simulink library "PAYLOAD_MASTER"  (Simulink 8.8)
settings: Solver=ode45  StartTime=0.0  StopTime=10.0  RelTol=1e-3  EnableMultiTasking=on
libraries: cdsEpicsOut x123, cdsFilt x55, cdsTP x42, cdsFiltCtrl x33, cdsEpicsIn x31, cdsMuxMatrix x17, cdsEpicsBinIn x17, VIS_LIB x13, PAYLOAD_MASTER x13, cdsRms x8, simulink x6, cdsEpicsStringIn x6
(part 3 of 12)

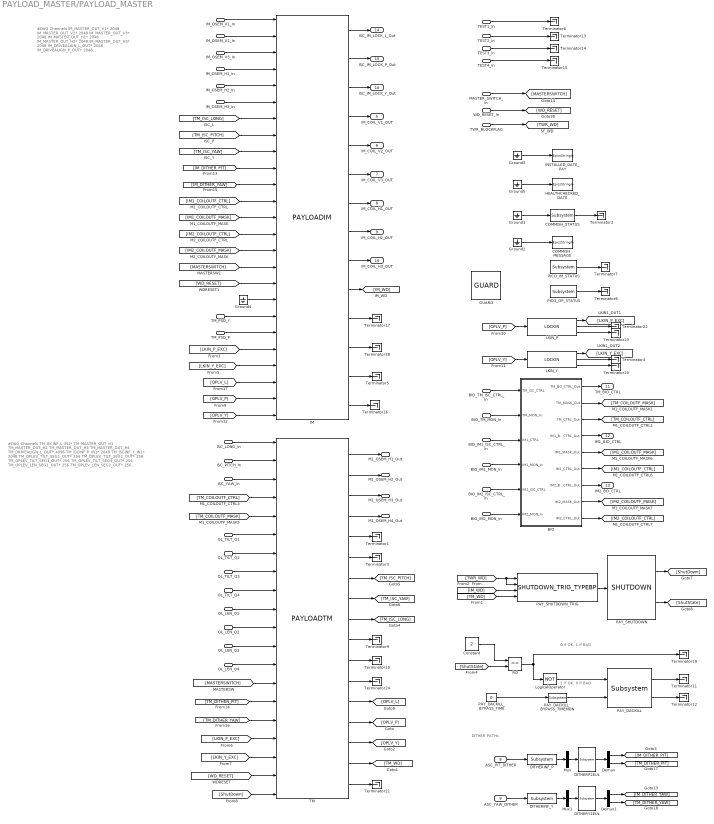
== system PAYLOAD_MASTER/PAYLOAD_MASTER ==
  note: 0 if OK, 1 if BAD
  note: 1 if OK, 0 if BAD
  note: #DAQ Channels
      | IM_MASTER_OUT_V1* 2048
      | IM_MASTER_OUT_V2* 2048
      | IM_MASTER_OUT_V3* 2048
      | IM_MASTER_OUT_H1* 2048
      | IM_MASTER_OUT_H2* 2048
      | IM_MASTER_OUT_H3* 2048
      | IM_DRIVEALIGN_L_OUT* 2048
      | IM_DRIVEALIGN_P_OUT* 2048
      | IM_DRIVEALIGN_Y_OUT* 2048
      | IM_CAL_LINE_OUT* 512
      | IM_OLDAMP_P_OUT* 256
      | IM_OLDAMP_Y_OUT* 256
      | IM_OSEMINF_V1_OUT* 256
      | IM_OSEMINF_V2_OUT* 256
      | IM_OSEMINF_V3_OUT* 256
      | IM_OSEMINF_H1_OUT* 256
      | IM_OSEMINF_H2_OUT* 256
      | IM_OSEMINF_H3_OUT* 256
  note: #DAQ Channels
      | TM_ISCINF_L_IN1*
      | TM_MASTER_OUT_H1
      | TM_MASTER_OUT_H2
      | TM_MASTER_OUT_H3
      | TM_MASTER_OUT_H4
      |
      | TM_DRIVEALIGN_L_OUT* 4096
      |
      | TM_ISCINF_P_IN1* 2048
      | TM_ISCINF_Y_IN1* 2048
      |
      | TM_OPLEV_TILT_SEG1_OUT* 256
      | TM_OPLEV_TILT_SEG2_OUT* 256
      | TM_OPLEV_TILT_SEG3_OUT* 256
      | TM_OPLEV_TILT_SEG4_OUT* 256
      | TM_OPLEV_LEN_SEG1_OUT* 256
      | TM_OPLEV_LEN_SEG2_OUT* 256
      | TM_OPLEV_LEN_SEG3_OUT* 256
      | TM_OPLEV_LEN_SEG4_OUT* 256
      |
      | TM_OPLEV_TILT_PIT_OUT* 256
      | TM_OPLEV_TILT_YAW_OUT* 256
      | TM_OPLEV_TILT_SUM_OUT* 256
      | TM_OPLEV_LEN_PIT_OUT* 256
      | TM_OPLEV_LEN_YAW_OUT* 256
      | TM_OPLEV_LEN_SUM_OUT* 256
  note: DITHER PATHs
  ISC_LONG_In : Inport
  ISC_PITCH_In : Inport  Port=2
  ISC_YAW_In : Inport  Port=3
  OL_TILT_Q1 : Inport  Port=4
  OL_TILT_Q2 : Inport  Port=5
  OL_TILT_Q3 : Inport  Port=6
  OL_TILT_Q4 : Inport  Port=7
  ASC_PIT_DITHER : Inport  Port=8
  ASC_YAW_DITHER : Inport  Port=9
  IM_OSEM_V1_In : Inport  Port=10
  IM_OSEM_V2_In : Inport  Port=11
  IM_OSEM_V3_In : Inport  Port=12
  IM_OSEM_H1_In : Inport  Port=13
  IM_OSEM_H2_In : Inport  Port=14
  IM_OSEM_H3_In : Inport  Port=15
  TEST1_In : Inport  Port=16
  TEST2_In : Inport  Port=17
  TEST3_In : Inport  Port=18
  TEST4_In : Inport  Port=19
  OL_LEN_Q1 : Inport  Port=20
  OL_LEN_Q2 : Inport  Port=21
  OL_LEN_Q3 : Inport  Port=22
  OL_LEN_Q4 : Inport  Port=23
  BIO_TM_ISC_CTRL_In : Inport  Port=24
  BIO_IM1_ISC_CTRL_In : Inport  Port=25
  BIO_IM2_ISC_CTRL_In : Inport  Port=26
  BIO_TM_MON_In : Inport  Port=27
  BIO_IM1_MON_In : Inport  Port=28
  BIO_IM2_MON_In : Inport  Port=29
  TM_PSD_P : Inport  Port=30
  TM_PSD_Y : Inport  Port=31
  MASTER_SWITCH_In : Inport  Port=32
  WD_RESET_In : Inport  Port=33
  TWR_BLOCKFLAG : Inport  Port=34
  BIO : Subsystem
  COMMISH_MESSAGE : cdsEpicsStringIn/EpicsStringIn  Tag=cdsEpicsStringIn  Description=cdsEpicsStringIn
      settings: AttributesFormatString=%<Tag>
  COMMISH_STATUS : cdsEpicsBinIn/Subsystem  Tag=cdsEpicsBinIn  Description=|
      | Purpose:                                                                            
      | Create an EPICS binary (0 or 1) input channel to the FE realtime controls.          
      |                                                                                     
      | Operation:                                                                          
      | Outputs value from an EPICS ai record. Value is binary input (bi Epics record type).
      |                                                                                     
      | Usage:                                                                              
      | Name the part with the desired EPICS channel name.
      settings: AttributesFormatString=%<Tag>
  Constant : Constant  Value=2
  DITHERINF_P : cdsFilt/Subsystem  Tag=cdsFilt  Description=|
      | Purpose:                                                                                                                                                                                                                                  
      | Standard CDS IIR filter module.                                                                                                                                                                                                           
      |                                                                                                                                                                                                                                           
      | Operation:                                                                                                                                                                                                                                
      | Consists of 10 second order section IIR filters, plus a ramped gain stage. In FE code, also provides pre-defined test points and excitation channel inputs. The filter coefficients are defined in the LIGO system using the 'foton' tool.
      |                                                                                                                                                                                                                                           
      | Usage:                                                                                                                                                                                                                                    
      | Name the part with the desired filter module name.
      settings: AttributesFormatString=%<Tag>
  DITHERINF_Y : cdsFilt/Subsystem  Tag=cdsFilt  Description=|
      | Purpose:                                                                                                                                                                                                                                  
      | Standard CDS IIR filter module.                                                                                                                                                                                                           
      |                                                                                                                                                                                                                                           
      | Operation:                                                                                                                                                                                                                                
      | Consists of 10 second order section IIR filters, plus a ramped gain stage. In FE code, also provides pre-defined test points and excitation channel inputs. The filter coefficients are defined in the LIGO system using the 'foton' tool.
      |                                                                                                                                                                                                                                           
      | Usage:                                                                                                                                                                                                                                    
      | Name the part with the desired filter module name.
      settings: AttributesFormatString=%<Tag>
  DITHERP2EUL : cdsMuxMatrix/Subsystem  Tag=cdsMuxMatrix  Description=Any size matrix. Inputs and outputs must be connected using Mux and Demux parts.
      settings: AttributesFormatString=%<Tag>
  DITHERY2EUL : cdsMuxMatrix/Subsystem  Tag=cdsMuxMatrix  Description=Any size matrix. Inputs and outputs must be connected using Mux and Demux parts.
      settings: AttributesFormatString=%<Tag>
  Demux : Demux  Outputs=2
  Demux1 : Demux  Outputs=2
  GUARD : ISC_common/GUARD
  Ground{1..5} (5 alike) : Ground
  HEALTHCHECKED_DATE : cdsEpicsStringIn/EpicsStringIn  Tag=cdsEpicsStringIn  Description=cdsEpicsStringIn
      settings: AttributesFormatString=%<Tag>
  IM : PAYLOAD_MASTER/PAYLOADIM  Description=SIXOSEMSTAGE_FACE_MASTER
  INSTALLED_DATE_PAY : cdsEpicsStringIn/EpicsStringIn  Tag=cdsEpicsStringIn  Description=cdsEpicsStringIn
      settings: AttributesFormatString=%<Tag>
  LKIN_P : lockin/LOCKIN  Description=ADL=LOCKIN.adl
      settings: AttributesFormatString=%<Tag>
  LKIN_Y : lockin/LOCKIN  Description=ADL=LOCKIN.adl
      settings: AttributesFormatString=%<Tag>
  LogicalOperator : Logic  Operator=NOT  AllPortsSameDT=off  OutDataTypeStr=boolean
  Mux : Mux  Inputs=1
  Mux1 : Mux  Inputs=1
  PAY_DACKILL : cdsDacKill/Subsystem  Description=cdsDacKill
      settings: AttributesFormatString=%<Description>
  PAY_DACKILL_BYPASS_TIME : Constant  Value=0
  PAY_DACKILL_BYPASS_TIMEMON : cdsEpicsOut/Subsystem  Tag=cdsEpicsOutput  Description=|
      | Purpose:                                          
      | Output a FE signal to an EPICS channel.           
      |                                                   
      | Operation:                                        
      | Takes input value and passes it to EPICS record.  
      |                                                   
      | Usage:                                            
      | Name the part with the desired EPICS rrecord name.
      settings: AttributesFormatString=%<Tag>
  PAY_SHUTDOWN : SHUTDOWN/SHUTDOWN
  PAY_SHUTDOWN_TRIG : VIS_LIB/SHUTDOWN_TRIG_TYPEBP
  PICO_IM_STATUS : cdsEpicsIn/Subsystem  Tag=cdsEpicsIn  Description=|
      | Purpose:                                                                              
      | Create an EPICS input channel connection to the FE realtime controls.                 
      |                                                                                       
      | Operation:                                                                            
      | Outputs value from an EPICS ai record. Value is floating point with a precision of 3..
      |                                                                                       
      | Usage:                                                                                
      | Name the part with the desired EPICS channel name.
      settings: AttributesFormatString=%<Tag>
  PICO_OP_STATUS : cdsEpicsIn/Subsystem  Tag=cdsEpicsIn  Description=|
      | Purpose:                                                                              
      | Create an EPICS input channel connection to the FE realtime controls.                 
      |                                                                                       
      | Operation:                                                                            
      | Outputs value from an EPICS ai record. Value is floating point with a precision of 3..
      |                                                                                       
      | Usage:                                                                                
      | Name the part with the desired EPICS channel name.
      settings: AttributesFormatString=%<Tag>
  RO : RelationalOperator  Operator===  OutDataTypeStr=boolean  RndMeth=Nearest
  TM : PAYLOAD_MASTER/PAYLOADTM
  Terminator{1..24} (24 alike) : Terminator
  M1_OSEM_H1_Out : Outport
  M1_OSEM_H2_Out : Outport  Port=2
  M1_OSEM_H3_Out : Outport  Port=3
  M1_OSEM_H4_Out : Outport  Port=4
  IM_COIL_V1_OUT : Outport  Port=5
  IM_COIL_V2_OUT : Outport  Port=6
  IM_COIL_V3_OUT : Outport  Port=7
  IM_COIL_H1_OUT : Outport  Port=8
  IM_COIL_H2_OUT : Outport  Port=9
  IM_COIL_H3_OUT : Outport  Port=10
  TM_BIO_CTRL : Outport  Port=11
  IM1_BIO_CTRL : Outport  Port=12
  IM2_BO_CTRL : Outport  Port=13
  ISC_IM_LOCK_L_Out : Outport  Port=14
  ISC_IM_LOCK_P_Out : Outport  Port=15
  ISC_IM_LOCK_Y_Out : Outport  Port=16
  wires:
  TM_PSD_Y/1 -> IM/19
  TM_PSD_P/1 -> IM/20
  TWR_BLOCKFLAG/1 -> [TWR_WD]
  WD_RESET_In/1 -> [WD_RESET]
  MASTER_SWITCH_In/1 -> [MASTERSWITCH]
  [TM_COILOUTF_MASK] -> TM/5
  [TM_COILOUTF_CTRL] -> TM/4
  [WD_RESET] -> TM/19
  TM/5 -> Terminator1/1
  [MASTERSWITCH] -> TM/14
  OL_TILT_Q4/1 -> TM/9
  ISC_YAW_In/1 -> TM/3
  ISC_PITCH_In/1 -> TM/2
  OL_TILT_Q3/1 -> TM/8
  OL_TILT_Q2/1 -> TM/7
  OL_TILT_Q1/1 -> TM/6
  TM/4 -> M1_OSEM_H4_Out/1
  TM/3 -> M1_OSEM_H3_Out/1
  TM/2 -> M1_OSEM_H2_Out/1
  ISC_LONG_In/1 -> TM/1
  Ground2/1 -> COMMISH_MESSAGE/1
  COMMISH_STATUS/1 -> Terminator2/1
  Ground1/1 -> COMMISH_STATUS/1
  [TM_DITHER_PIT] -> TM/15
  [TM_DITHER_YAW] -> TM/16
  [TM_ISC_LONG] -> IM/7
  [TM_ISC_PITCH] -> IM/8
  [TM_ISC_YAW] -> IM/9
  IM/10 -> [IM_WD]
  IM/11 -> Terminator17/1
  IM/12 -> Terminator18/1
  IM_OSEM_V3_In/1 -> IM/3
  IM_OSEM_V2_In/1 -> IM/2
  IM_OSEM_V1_In/1 -> IM/1
  IM_OSEM_H3_In/1 -> IM/6
  IM_OSEM_H2_In/1 -> IM/5
  IM_OSEM_H1_In/1 -> IM/4
  IM/4 -> IM_COIL_V1_OUT/1
  IM/5 -> IM_COIL_V2_OUT/1
  IM/6 -> IM_COIL_V3_OUT/1
  IM/7 -> IM_COIL_H1_OUT/1
  IM/8 -> IM_COIL_H2_OUT/1
  IM/9 -> IM_COIL_H3_OUT/1
  TEST3_In/1 -> Terminator14/1
  TEST2_In/1 -> Terminator13/1
  TEST1_In/1 -> Terminator6/1
  TEST4_In/1 -> Terminator15/1
  TM/1 -> M1_OSEM_H1_Out/1
  [TM_WD] -> PAY_SHUTDOWN_TRIG/4
  LogicalOperator/1 -> PAY_DACKILL/1
  PAY_DACKILL_BYPASS_TIMEMON/1 -> PAY_DACKILL/2
  PAY_DACKILL_BYPASS_TIME/1 -> PAY_DACKILL_BYPASS_TIMEMON/1
  PAY_DACKILL/1 -> Terminator11/1
  PAY_DACKILL/2 -> Terminator12/1
  [IM_WD] -> PAY_SHUTDOWN_TRIG/3
  [IM1_COILOUTF_CTRL] -> IM/12
  [IM_DITHER_PIT] -> IM/10
  [IM_DITHER_YAW] -> IM/11
  [IM1_COILOUTF_MASK] -> IM/13
  [TWR_WD] -> PAY_SHUTDOWN_TRIG/1, PAY_SHUTDOWN_TRIG/2
  OL_LEN_Q4/1 -> TM/13
  OL_LEN_Q3/1 -> TM/12
  OL_LEN_Q2/1 -> TM/11
  OL_LEN_Q1/1 -> TM/10
  BIO/3(TM_CTRL_Out) -> [TM_COILOUTF_CTRL]
  BIO/2(TM_MASK_Out) -> [TM_COILOUTF_MASK]
  BIO/6(IM1_CTRL_Out) -> [IM1_COILOUTF_CTRL]
  BIO/5(IM1_MASK_Out) -> [IM1_COILOUTF_MASK]
  BIO/7(IM2_BO_CTRL_Out) -> IM2_BO_CTRL/1
  BIO/4(IM1_BO_CTRL_Out) -> IM1_BIO_CTRL/1
  BIO/1(TM_BO_CTRL_Out) -> TM_BIO_CTRL/1
  BIO_IM2_MON_In/1 -> BIO/6(IM2_MON_In)
  BIO_IM2_ISC_CTRL_In/1 -> BIO/5(IM2_ISC_CTRL)
  BIO_IM1_MON_In/1 -> BIO/4(IM1_MON_In)
  BIO_IM1_ISC_CTRL_In/1 -> BIO/3(IM1_CTRL)
  BIO_TM_MON_In/1 -> BIO/2(TM_MON_In)
  BIO_TM_ISC_CTRL_In/1 -> BIO/1(TM_ISC_CTRL)
  BIO/8(IM2_MASK_Out) -> [IM2_COILOUTF_MASK]
  BIO/9(IM2_CTRL_Out) -> [IM2_COILOUTF_CTRL]
  [MASTERSWITCH] -> IM/16
  [WD_RESET] -> IM/17
  [IM2_COILOUTF_CTRL] -> IM/14
  [IM2_COILOUTF_MASK] -> IM/15
  TM/9 -> [TM_ISC_LONG]
  TM/7 -> [TM_ISC_PITCH]
  TM/8 -> [TM_ISC_YAW]
  PAY_SHUTDOWN_TRIG/1 -> PAY_SHUTDOWN/1
  PAY_SHUTDOWN/1 -> [ShutDown]
  PAY_SHUTDOWN/2 -> [ShutState]
  RO/1 -> Terminator19/1, LogicalOperator/1
  Constant/1 -> RO/1
  [ShutState] -> RO/2
  [ShutDown] -> TM/20
  IM/1 -> ISC_IM_LOCK_L_Out/1
  IM/2 -> ISC_IM_LOCK_P_Out/1
  IM/3 -> ISC_IM_LOCK_Y_Out/1
  Ground3/1 -> INSTALLED_DATE_PAY/1
  Ground5/1 -> HEALTHCHECKED_DATE/1
  PICO_OP_STATUS/1 -> Terminator8/1
  PICO_IM_STATUS/1 -> Terminator7/1
  Ground4/1 -> IM/18
  [LKIN_P_EXC] -> IM/21
  [LKIN_Y_EXC] -> IM/22
  IM/13 -> Terminator5/1
  TM/10 -> Terminator9/1
  TM/6 -> Terminator3/1
  TM/11 -> Terminator10/1
  [LKIN_P_EXC] -> TM/17
  [LKIN_Y_EXC] -> TM/18
  [OPLV_P] -> LKIN_P/1
  LKIN_P/2 -> Terminator22/1
  LKIN_P/3 -> Terminator23/1
  LKIN_P/1 -> [LKIN_P_EXC]
  LKIN_Y/1 -> [LKIN_Y_EXC]
  [OPLV_Y] -> LKIN_Y/1
  LKIN_Y/2 -> Terminator4/1
  LKIN_Y/3 -> Terminator20/1
  IM/14 -> Terminator16/1
  ASC_YAW_DITHER/1 -> DITHERINF_Y/1
  ASC_PIT_DITHER/1 -> DITHERINF_P/1
  DITHERINF_P/1 -> Mux/1
  Mux/1 -> DITHERP2EUL/1
  DITHERP2EUL/1 -> Demux/1
  Demux/1 -> [IM_DITHER_PIT]
  Mux1/1 -> DITHERY2EUL/1
  DITHERY2EUL/1 -> Demux1/1
  Demux1/1 -> [IM_DITHER_YAW]
  DITHERINF_Y/1 -> Mux1/1
  Demux/2 -> [TM_DITHER_PIT]
  Demux1/2 -> [TM_DITHER_YAW]
  TM/14 -> [OPLV_P]
  TM/15 -> [OPLV_Y]
  TM/16 -> [TM_WD]
  TM/17 -> Terminator21/1
  TM/13 -> [OPLV_L]
  TM/12 -> Terminator24/1
  [OPLV_P] -> IM/24
  [OPLV_Y] -> IM/25
  [OPLV_L] -> IM/23

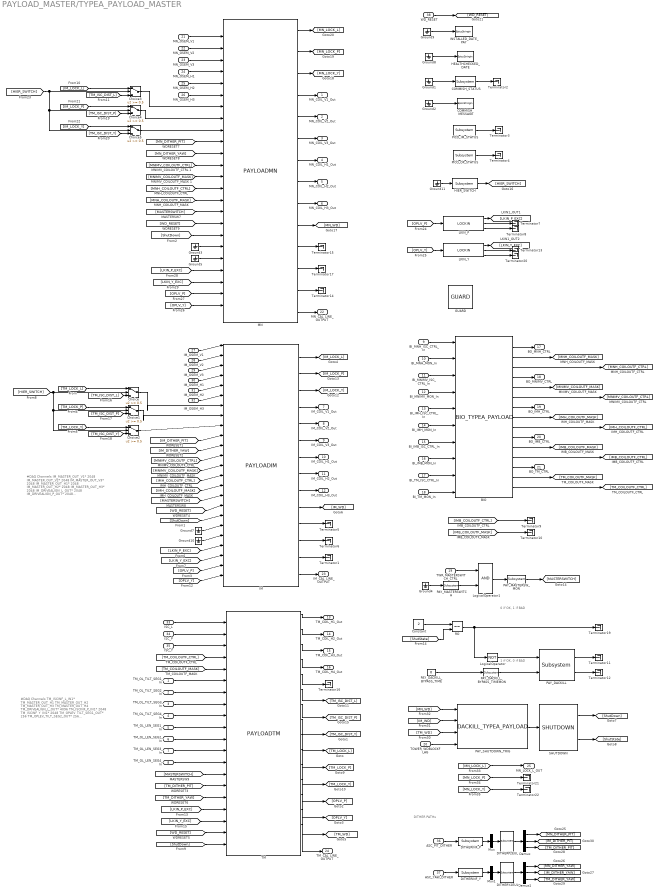
== system PAYLOAD_MASTER/TYPEA_PAYLOAD_MASTER ==
  note: 1 if OK, 0 if BAD
  note: 0 if OK, 1 if BAD
  note: DITHER PATHs
  note: #DAQ Channels
      | IM_MASTER_OUT_V1* 2048
      | IM_MASTER_OUT_V2* 2048
      | IM_MASTER_OUT_V3* 2048
      | IM_MASTER_OUT_H1* 2048
      | IM_MASTER_OUT_H2* 2048
      | IM_MASTER_OUT_H3* 2048
      | IM_DRIVEALIGN_L_OUT* 2048
      | IM_DRIVEALIGN_P_OUT* 2048
      | IM_DRIVEALIGN_Y_OUT* 2048
      | IM_CAL_LINE_OUT* 512
      | IM_OLDAMP_P_OUT* 256
      | IM_OLDAMP_Y_OUT* 256
      | IM_OSEMINF_V1_OUT* 256
      | IM_OSEMINF_V2_OUT* 256
      | IM_OSEMINF_V3_OUT* 256
      | IM_OSEMINF_H1_OUT* 256
      | IM_OSEMINF_H2_OUT* 256
      | IM_OSEMINF_H3_OUT* 256
  note: #DAQ Channels
      | TM_ISCINF_L_IN1*
      | TM_MASTER_OUT_H1
      | TM_MASTER_OUT_H2
      | TM_MASTER_OUT_H3
      | TM_MASTER_OUT_H4
      |
      | TM_DRIVEALIGN_L_OUT* 4096
      |
      | TM_ISCINF_P_IN1* 2048
      | TM_ISCINF_Y_IN1* 2048
      |
      | TM_OPLEV_TILT_SEG1_OUT* 256
      | TM_OPLEV_TILT_SEG2_OUT* 256
      | TM_OPLEV_TILT_SEG3_OUT* 256
      | TM_OPLEV_TILT_SEG4_OUT* 256
      | TM_OPLEV_LEN_SEG1_OUT* 256
      | TM_OPLEV_LEN_SEG2_OUT* 256
      | TM_OPLEV_LEN_SEG3_OUT* 256
      | TM_OPLEV_LEN_SEG4_OUT* 256
      |
      | TM_OPLEV_TILT_PIT_OUT* 256
      | TM_OPLEV_TILT_YAW_OUT* 256
      | TM_OPLEV_TILT_SUM_OUT* 256
      | TM_OPLEV_LEN_PIT_OUT* 256
      | TM_OPLEV_LEN_YAW_OUT* 256
      | TM_OPLEV_LEN_SUM_OUT* 256
  TM_OL_TILT_SEG1_In : Inport
  TM_OL_TILT_SEG2_In : Inport  Port=2
  TM_OL_TILT_SEG3_In : Inport  Port=3
  TM_OL_TILT_SEG4_In : Inport  Port=4
  TM_OL_LEN_SEG1_In : Inport  Port=5
  TM_OL_LEN_SEG2_In : Inport  Port=6
  TM_OL_LEN_SEG3_In : Inport  Port=7
  TM_OL_LEN_SEG4_In : Inport  Port=8
  BI_MNH_ISC_CTRL_In : Inport  Port=9
  BI_MNH_MON_In : Inport  Port=10
  BI_MNIMV_ISC_CTRL_In : Inport  Port=11
  BI_MNIMV_MON_In : Inport  Port=12
  BI_IMH_ISC_CTRL_In : Inport  Port=13
  BI_IMH_MON_In : Inport  Port=14
  BI_IMB_ISC_CTRL_In : Inport  Port=15
  BI_IMB_MON_In : Inport  Port=16
  BI_TM_ISC_CTRL_In : Inport  Port=17
  BI_TM_MON_In : Inport  Port=18
  TWR_MASTERSWITCH_CTRL : Inport  Port=19
  TOWER_WDBLOCKFLAG : Inport  Port=20
  MN_OSEM_V1 : Inport  Port=21
  MN_OSEM_V2 : Inport  Port=22
  MN_OSEM_V3 : Inport  Port=23
  MN_OSEM_H1 : Inport  Port=24
  MN_OSEM_H2 : Inport  Port=25
  MN_OSEM_H3 : Inport  Port=26
  IM_OSEM_V1 : Inport  Port=27
  IM_OSEM_V2 : Inport  Port=28
  IM_OSEM_V3 : Inport  Port=29
  IM_OSEM_H1 : Inport  Port=30
  IM_OSEM_H2 : Inport  Port=31
  IM_OSEM_H3 : Inport  Port=32
  ISC_L : Inport  Port=33
  ISC_P : Inport  Port=34
  ISC_Y : Inport  Port=35
  ASC_PIT_DITHER : Inport  Port=36
  ASC_YAW_DITHER : Inport  Port=37
  WD_RESET : Inport  Port=38
  BIO : VIS_LIB/BIO_TYPEA_PAYLOAD
  COMMISH_MESSAGE : cdsEpicsStringIn/EpicsStringIn  Tag=cdsEpicsStringIn  Description=cdsEpicsStringIn
      settings: AttributesFormatString=%<Tag>
  COMMISH_STATUS : cdsEpicsBinIn/Subsystem  Tag=cdsEpicsBinIn  Description=|
      | Purpose:                                                                            
      | Create an EPICS binary (0 or 1) input channel to the FE realtime controls.          
      |                                                                                     
      | Operation:                                                                          
      | Outputs value from an EPICS ai record. Value is binary input (bi Epics record type).
      |                                                                                     
      | Usage:                                                                              
      | Name the part with the desired EPICS channel name.
      settings: AttributesFormatString=%<Tag>
  Choice{,1..5} (6 alike) : Switch  Threshold=0.5
  Constant : Constant  Value=2
  DITHERINF_P : cdsFilt/Subsystem  Tag=cdsFilt  Description=|
      | Purpose:                                                                                                                                                                                                                                  
      | Standard CDS IIR filter module.                                                                                                                                                                                                           
      |                                                                                                                                                                                                                                           
      | Operation:                                                                                                                                                                                                                                
      | Consists of 10 second order section IIR filters, plus a ramped gain stage. In FE code, also provides pre-defined test points and excitation channel inputs. The filter coefficients are defined in the LIGO system using the 'foton' tool.
      |                                                                                                                                                                                                                                           
      | Usage:                                                                                                                                                                                                                                    
      | Name the part with the desired filter module name.
      settings: AttributesFormatString=%<Tag>
  DITHERINF_Y : cdsFilt/Subsystem  Tag=cdsFilt  Description=|
      | Purpose:                                                                                                                                                                                                                                  
      | Standard CDS IIR filter module.                                                                                                                                                                                                           
      |                                                                                                                                                                                                                                           
      | Operation:                                                                                                                                                                                                                                
      | Consists of 10 second order section IIR filters, plus a ramped gain stage. In FE code, also provides pre-defined test points and excitation channel inputs. The filter coefficients are defined in the LIGO system using the 'foton' tool.
      |                                                                                                                                                                                                                                           
      | Usage:                                                                                                                                                                                                                                    
      | Name the part with the desired filter module name.
      settings: AttributesFormatString=%<Tag>
  DITHERP2EUL : cdsMuxMatrix/Subsystem  Tag=cdsMuxMatrix  Description=Any size matrix. Inputs and outputs must be connected using Mux and Demux parts.
      settings: AttributesFormatString=%<Tag>
  DITHERY2EUL : cdsMuxMatrix/Subsystem  Tag=cdsMuxMatrix  Description=Any size matrix. Inputs and outputs must be connected using Mux and Demux parts.
      settings: AttributesFormatString=%<Tag>
  Demux : Demux  Outputs=3
  Demux1 : Demux  Outputs=3
  GUARD : ISC_common/GUARD
  Ground{1..5,7..11} (10 alike) : Ground
  HEALTHCHECKED_DATE : cdsEpicsStringIn/EpicsStringIn  Tag=cdsEpicsStringIn  Description=cdsEpicsStringIn
      settings: AttributesFormatString=%<Tag>
  HIER_SWITCH : cdsEpicsBinIn/Subsystem  Tag=cdsEpicsBinIn  Description=|
      | Purpose:                                                                            
      | Create an EPICS binary (0 or 1) input channel to the FE realtime controls.          
      |                                                                                     
      | Operation:                                                                          
      | Outputs value from an EPICS ai record. Value is binary input (bi Epics record type).
      |                                                                                     
      | Usage:                                                                              
      | Name the part with the desired EPICS channel name.
      settings: AttributesFormatString=%<Tag>
  IM : PAYLOAD_MASTER/PAYLOADIM  Description=SIXOSEMSTAGE_FACE_MASTER
  INSTALLED_DATE_PAY : cdsEpicsStringIn/EpicsStringIn  Tag=cdsEpicsStringIn  Description=cdsEpicsStringIn
      settings: AttributesFormatString=%<Tag>
  LKIN_P : lockin/LOCKIN  Description=ADL=LOCKIN.adl
      settings: AttributesFormatString=%<Tag>
  LKIN_Y : lockin/LOCKIN  Description=ADL=LOCKIN.adl
      settings: AttributesFormatString=%<Tag>
  LogicalOperator : Logic  Operator=NOT  AllPortsSameDT=off  OutDataTypeStr=boolean
  LogicalOperator1 : Logic  AllPortsSameDT=off  OutDataTypeStr=boolean
  MN : PAYLOAD_MASTER/PAYLOADMN  Description=SIXOSEMSTAGE_FACE_MASTER
  Mux : Mux  Inputs=1
  Mux1 : Mux  Inputs=1
  PAY_DACKILL : cdsDacKill/Subsystem  Description=cdsDacKill
      settings: AttributesFormatString=%<Description>
  PAY_DACKILL_BYPASS_TIME : Constant  Value=0
  PAY_DACKILL_BYPASS_TIMEMON : cdsEpicsOut/Subsystem  Tag=cdsEpicsOutput  Description=|
      | Purpose:                                          
      | Output a FE signal to an EPICS channel.           
      |                                                   
      | Operation:                                        
      | Takes input value and passes it to EPICS record.  
      |                                                   
      | Usage:                                            
      | Name the part with the desired EPICS rrecord name.
      settings: AttributesFormatString=%<Tag>
  PAY_MASTERSWITCH : cdsEpicsBinIn/Subsystem  Tag=cdsEpicsBinIn  Description=|
      | Purpose:                                                                            
      | Create an EPICS binary (0 or 1) input channel to the FE realtime controls.          
      |                                                                                     
      | Operation:                                                                          
      | Outputs value from an EPICS ai record. Value is binary input (bi Epics record type).
      |                                                                                     
      | Usage:                                                                              
      | Name the part with the desired EPICS channel name.
      settings: AttributesFormatString=%<Tag>
  PAY_MASTERSW_MON : cdsEpicsOut/Subsystem  Tag=cdsEpicsOutput  Description=|
      | Purpose:                                          
      | Output a FE signal to an EPICS channel.           
      |                                                   
      | Operation:                                        
      | Takes input value and passes it to EPICS record.  
      |                                                   
      | Usage:                                            
      | Name the part with the desired EPICS rrecord name.
      settings: AttributesFormatString=%<Tag>
  PAY_SHUTDOWN_TRIG : VIS_LIB/DACKILL_TYPEA_PAYLOAD
  PICO_IM_STATUS : cdsEpicsIn/Subsystem  Tag=cdsEpicsIn  Description=|
      | Purpose:                                                                              
      | Create an EPICS input channel connection to the FE realtime controls.                 
      |                                                                                       
      | Operation:                                                                            
      | Outputs value from an EPICS ai record. Value is floating point with a precision of 3..
      |                                                                                       
      | Usage:                                                                                
      | Name the part with the desired EPICS channel name.
      settings: AttributesFormatString=%<Tag>
  PICO_OP_STATUS : cdsEpicsIn/Subsystem  Tag=cdsEpicsIn  Description=|
      | Purpose:                                                                              
      | Create an EPICS input channel connection to the FE realtime controls.                 
      |                                                                                       
      | Operation:                                                                            
      | Outputs value from an EPICS ai record. Value is floating point with a precision of 3..
      |                                                                                       
      | Usage:                                                                                
      | Name the part with the desired EPICS channel name.
      settings: AttributesFormatString=%<Tag>
  RO : RelationalOperator  Operator===  OutDataTypeStr=boolean  RndMeth=Nearest
  SHUTDOWN : SHUTDOWN/SHUTDOWN
  TM : PAYLOAD_MASTER/PAYLOADTM
  Terminator{1..17,19..22} (21 alike) : Terminator
  MN_COIL_V1_Out : Outport
  MN_COIL_V2_Out : Outport  Port=2
  MN_COIL_V3_Out : Outport  Port=3
  MN_COIL_H1_Out : Outport  Port=4
  MN_COIL_H2_Out : Outport  Port=5
  MN_COIL_H3_Out : Outport  Port=6
  IM_COIL_V1_Out : Outport  Port=7
  IM_COIL_V2_Out : Outport  Port=8
  IM_COIL_V3_Out : Outport  Port=9
  IM_COIL_H1_Out : Outport  Port=10
  IM_COIL_H2_Out : Outport  Port=11
  IM_COIL_H3_Out : Outport  Port=12
  TM_COIL_H1_Out : Outport  Port=13
  TM_COIL_H2_Out : Outport  Port=14
  TM_COIL_H3_Out : Outport  Port=15
  TM_COIL_H4_Out : Outport  Port=16
  BO_MNH_CTRL : Outport  Port=17
  BO_MNIMV_CTRL : Outport  Port=18
  BO_IMH_CTRL : Outport  Port=19
  BO_IMB_CTRL : Outport  Port=20
  BO_TM_CTRL : Outport  Port=21
  MN_CAL_LINE_OUTPUT : Outport  Port=22
  IM_CAL_LINE_OUTPUT : Outport  Port=23
  TM_CAL_LINE_OUTPUT : Outport  Port=24
  MN_LOCK_L_OUT : Outport  Port=25
  wires:
  PICO_OP_STATUS/1 -> Terminator4/1
  PICO_IM_STATUS/1 -> Terminator3/1
  Ground9/1 -> INSTALLED_DATE_PAY/1
  Ground8/1 -> HEALTHCHECKED_DATE/1
  [TM_WD] -> PAY_SHUTDOWN_TRIG/3
  [IM_WD] -> PAY_SHUTDOWN_TRIG/2
  [MN_WD] -> PAY_SHUTDOWN_TRIG/1
  [TM_COILOUTF_CTRL] -> TM/4
  [ShutDown] -> MN/18
  [ShutDown] -> IM/18
  [MNIMV_COILOUTF_MASK] -> MN/13
  [MNIMV_COILOUTF_CTRL] -> MN/12
  [MNH_COILOUTF_MASK] -> MN/15
  [MNH_COILOUTF_CTRL] -> MN/14
  [MASTERSWITCH] -> MN/16
  PAY_MASTERSW_MON/1 -> [MASTERSWITCH]
  LogicalOperator1/1 -> PAY_MASTERSW_MON/1
  TWR_MASTERSWITCH_CTRL/1 -> LogicalOperator1/1
  [MNIMV_COILOUTF_MASK] -> IM/13
  [MNIMV_COILOUTF_CTRL] -> IM/12
  [MASTERSWITCH] -> IM/16
  [IMH_COILOUTF_MASK] -> IM/15
  [IMH_COILOUTF_CTRL] -> IM/14
  RO/1 -> LogicalOperator/1, Terminator19/1
  [ShutState] -> RO/2
  Constant/1 -> RO/1
  SHUTDOWN/2 -> [ShutState]
  SHUTDOWN/1 -> [ShutDown]
  PAY_SHUTDOWN_TRIG/1 -> SHUTDOWN/1
  TOWER_WDBLOCKFLAG/1 -> PAY_SHUTDOWN_TRIG/4
  BI_TM_ISC_CTRL_In/1 -> BIO/9
  IM/9 -> IM_COIL_H3_Out/1
  BI_IMH_ISC_CTRL_In/1 -> BIO/5
  BI_MNIMV_ISC_CTRL_In/1 -> BIO/3
  BI_IMH_MON_In/1 -> BIO/6
  BI_MNIMV_MON_In/1 -> BIO/4
  BIO/9 -> [IMH_COILOUTF_CTRL]
  BIO/15 -> [TM_COILOUTF_CTRL]
  BIO/6 -> [MNIMV_COILOUTF_CTRL]
  BIO/12 -> [IMB_COILOUTF_CTRL]
  BIO/11 -> [IMB_COILOUTF_MASK]
  BIO/8 -> [IMH_COILOUTF_MASK]
  BIO/14 -> [TM_COILOUTF_MASK]
  BIO/5 -> [MNIMV_COILOUTF_MASK]
  BIO/4 -> BO_MNIMV_CTRL/1
  BIO/10 -> BO_IMB_CTRL/1
  BIO/13 -> BO_TM_CTRL/1
  BIO/7 -> BO_IMH_CTRL/1
  TM/4 -> TM_COIL_H4_Out/1
  TM/3 -> TM_COIL_H3_Out/1
  TM/2 -> TM_COIL_H2_Out/1
  TM/1 -> TM_COIL_H1_Out/1
  MN/4 -> MN_COIL_V1_Out/1
  MN/5 -> MN_COIL_V2_Out/1
  MN/6 -> MN_COIL_V3_Out/1
  MN/7 -> MN_COIL_H1_Out/1
  MN/8 -> MN_COIL_H2_Out/1
  MN/9 -> MN_COIL_H3_Out/1
  TM_OL_LEN_SEG3_In/1 -> TM/12
  TM_OL_LEN_SEG2_In/1 -> TM/11
  TM_OL_TILT_SEG4_In/1 -> TM/9
  TM_OL_LEN_SEG4_In/1 -> TM/13
  TM_OL_TILT_SEG3_In/1 -> TM/8
  TM_OL_TILT_SEG2_In/1 -> TM/7
  TM_OL_LEN_SEG1_In/1 -> TM/10
  TM_OL_TILT_SEG1_In/1 -> TM/6
  IM/8 -> IM_COIL_H2_Out/1
  IM/7 -> IM_COIL_H1_Out/1
  IM/6 -> IM_COIL_V3_Out/1
  IM/5 -> IM_COIL_V2_Out/1
  IM/4 -> IM_COIL_V1_Out/1
  BIO/3 -> [MNH_COILOUTF_CTRL]
  BIO/2 -> [MNH_COILOUTF_MASK]
  BIO/1 -> BO_MNH_CTRL/1
  BI_IMB_MON_In/1 -> BIO/8
  BI_TM_MON_In/1 -> BIO/10
  BI_IMB_ISC_CTRL_In/1 -> BIO/7
  BI_MNH_ISC_CTRL_In/1 -> BIO/1
  BI_MNH_MON_In/1 -> BIO/2
  [IMB_COILOUTF_MASK] -> Terminator10/1
  [IMB_COILOUTF_CTRL] -> Terminator9/1
  PAY_DACKILL/2 -> Terminator12/1
  PAY_DACKILL/1 -> Terminator11/1
  PAY_DACKILL_BYPASS_TIME/1 -> PAY_DACKILL_BYPASS_TIMEMON/1
  PAY_DACKILL_BYPASS_TIMEMON/1 -> PAY_DACKILL/2
  LogicalOperator/1 -> PAY_DACKILL/1
  Ground1/1 -> COMMISH_STATUS/1
  COMMISH_STATUS/1 -> Terminator2/1
  Ground2/1 -> COMMISH_MESSAGE/1
  PAY_MASTERSWITCH/1 -> LogicalOperator1/2
  Ground4/1 -> PAY_MASTERSWITCH/1
  [TM_COILOUTF_MASK] -> TM/5
  [MASTERSWITCH] -> TM/14
  [ShutDown] -> TM/20
  TM/9 -> [TM_LOCK_L]
  TM/10 -> [TM_LOCK_P]
  TM/11 -> [TM_LOCK_Y]
  TM/5 -> Terminator16/1
  TM/14 -> [TM_WD]
  TM/12 -> [OPLV_P]
  TM/13 -> [OPLV_Y]
  TM/6 -> [TM_ISC_DIST_L]
  TM/7 -> [TM_ISC_DIST_P]
  TM/8 -> [TM_ISC_DIST_Y]
  [TM_DITHER_PIT] -> TM/15
  [TM_DITHER_YAW] -> TM/16
  [LKIN_P_EXC] -> TM/17
  [LKIN_Y_EXC] -> TM/18
  [WD_RESET] -> TM/19
  IM/12 -> Terminator6/1
  IM/10 -> [IM_WD]
  IM/11 -> Terminator5/1
  IM/13 -> Terminator1/1
  [LKIN_P_EXC] -> IM/21
  [LKIN_Y_EXC] -> IM/22
  [OPLV_P] -> IM/23
  [OPLV_Y] -> IM/24
  Ground7/1 -> IM/19
  Ground10/1 -> IM/20
  [WD_RESET] -> IM/17
  [IM_DITHER_PIT] -> IM/10
  [IM_DITHER_YAW] -> IM/11
  [TM_LOCK_Y] -> Choice2/1
  [TM_LOCK_P] -> Choice1/1
  [TM_LOCK_L] -> Choice/1
  Ground11/1 -> HIER_SWITCH/1
  Choice2/1 -> IM/9
  Choice1/1 -> IM/8
  Choice/1 -> IM/7
  [TM_ISC_DIST_L] -> Choice/3
  [TM_ISC_DIST_P] -> Choice1/3
  [TM_ISC_DIST_Y] -> Choice2/3
  IM/1 -> [IM_LOCK_L]
  IM/2 -> [IM_LOCK_P]
  IM/3 -> [IM_LOCK_Y]
  ISC_L/1 -> TM/1
  ISC_P/1 -> TM/2
  ISC_Y/1 -> TM/3
  HIER_SWITCH/1 -> [HIER_SWITCH]
  [HIER_SWITCH] -> Choice2/2, Choice1/2, Choice/2
  [IM_LOCK_Y] -> Choice5/1
  [IM_LOCK_P] -> Choice4/1
  [IM_LOCK_L] -> Choice3/1
  Choice5/1 -> MN/9
  Choice4/1 -> MN/8
  Choice3/1 -> MN/7
  [TM_ISC_DIST_L] -> Choice3/3
  [TM_ISC_DIST_P] -> Choice4/3
  [TM_ISC_DIST_Y] -> Choice5/3
  [HIER_SWITCH] -> Choice5/2, Choice4/2, Choice3/2
  [OPLV_P] -> LKIN_P/1
  LKIN_P/2 -> Terminator7/1
  LKIN_P/3 -> Terminator8/1
  LKIN_P/1 -> [LKIN_P_EXC]
  LKIN_Y/1 -> [LKIN_Y_EXC]
  [OPLV_Y] -> LKIN_Y/1
  LKIN_Y/2 -> Terminator13/1
  LKIN_Y/3 -> Terminator20/1
  [LKIN_P_EXC] -> MN/21
  [LKIN_Y_EXC] -> MN/22
  [OPLV_P] -> MN/23
  [OPLV_Y] -> MN/24
  MN/12 -> Terminator17/1
  MN/10 -> [MN_WD]
  MN/11 -> Terminator15/1
  MN/13 -> Terminator14/1
  [MN_DITHER_PIT] -> MN/10
  [MN_DITHER_YAW] -> MN/11
  [WD_RESET] -> MN/17
  IM_OSEM_V1/1 -> IM/1
  IM_OSEM_V2/1 -> IM/2
  IM_OSEM_V3/1 -> IM/3
  IM_OSEM_H1/1 -> IM/4
  IM_OSEM_H2/1 -> IM/5
  IM_OSEM_H3/1 -> IM/6
  MN_OSEM_V1/1 -> MN/1
  MN_OSEM_V2/1 -> MN/2
  MN_OSEM_V3/1 -> MN/3
  MN_OSEM_H1/1 -> MN/4
  MN_OSEM_H2/1 -> MN/5
  MN_OSEM_H3/1 -> MN/6
  MN/1 -> [MN_LOCK_L]
  MN/2 -> [MN_LOCK_P]
  MN/3 -> [MN_LOCK_Y]
  [MN_LOCK_L] -> MN_LOCK_L_OUT/1
  [MN_LOCK_P] -> Terminator21/1
  [MN_LOCK_Y] -> Terminator22/1
  Ground3/1 -> MN/19
  Ground5/1 -> MN/20
  ASC_YAW_DITHER/1 -> DITHERINF_Y/1
  ASC_PIT_DITHER/1 -> DITHERINF_P/1
  DITHERINF_P/1 -> Mux/1
  Mux/1 -> DITHERP2EUL/1
  DITHERP2EUL/1 -> Demux/1
  Demux/1 -> [MN_DITHER_PIT]
  Mux1/1 -> DITHERY2EUL/1
  DITHERY2EUL/1 -> Demux1/1
  Demux1/1 -> [MN_DITHER_YAW]
  DITHERINF_Y/1 -> Mux1/1
  Demux/2 -> [IM_DITHER_PIT]
  Demux1/2 -> [IM_DITHER_YAW]
  Demux/3 -> [TM_DITHER_PIT]
  Demux1/3 -> [TM_DITHER_YAW]
  MN/14 -> MN_CAL_LINE_OUTPUT/1
  IM/14 -> IM_CAL_LINE_OUTPUT/1
  TM/15 -> TM_CAL_LINE_OUTPUT/1
  WD_RESET/1 -> [WD_RESET]

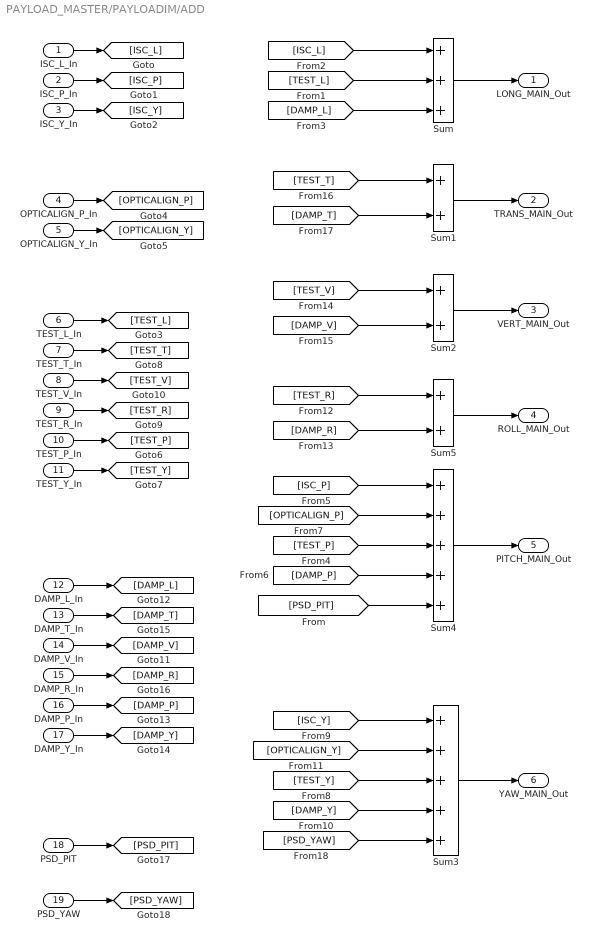
== system PAYLOAD_MASTER/PAYLOADIM/ADD ==
  ISC_L_In : Inport
  ISC_P_In : Inport  Port=2
  ISC_Y_In : Inport  Port=3
  OPTICALIGN_P_In : Inport  Port=4
  OPTICALIGN_Y_In : Inport  Port=5
  TEST_L_In : Inport  Port=6
  TEST_T_In : Inport  Port=7
  TEST_V_In : Inport  Port=8
  TEST_R_In : Inport  Port=9
  TEST_P_In : Inport  Port=10
  TEST_Y_In : Inport  Port=11
  DAMP_L_In : Inport  Port=12
  DAMP_T_In : Inport  Port=13
  DAMP_V_In : Inport  Port=14
  DAMP_R_In : Inport  Port=15
  DAMP_P_In : Inport  Port=16
  DAMP_Y_In : Inport  Port=17
  PSD_PIT : Inport  Port=18
  PSD_YAW : Inport  Port=19
  Sum : Sum  Inputs=+++
  Sum1 : Sum
  Sum2 : Sum
  Sum3 : Sum  Inputs=+++++
  Sum4 : Sum  Inputs=+++++
  Sum5 : Sum
  LONG_MAIN_Out : Outport
  TRANS_MAIN_Out : Outport  Port=2
  VERT_MAIN_Out : Outport  Port=3
  ROLL_MAIN_Out : Outport  Port=4
  PITCH_MAIN_Out : Outport  Port=5
  YAW_MAIN_Out : Outport  Port=6
  wires:
  [DAMP_V] -> Sum2/2
  [TEST_V] -> Sum2/1
  [DAMP_T] -> Sum1/2
  [TEST_T] -> Sum1/1
  [DAMP_R] -> Sum5/2
  [TEST_R] -> Sum5/1
  [DAMP_Y] -> Sum3/4
  [TEST_Y] -> Sum3/3
  [OPTICALIGN_Y] -> Sum3/2
  [ISC_Y] -> Sum3/1
  [DAMP_P] -> Sum4/4
  [TEST_P] -> Sum4/3
  [OPTICALIGN_P] -> Sum4/2
  [ISC_P] -> Sum4/1
  DAMP_Y_In/1 -> [DAMP_Y]
  DAMP_P_In/1 -> [DAMP_P]
  DAMP_R_In/1 -> [DAMP_R]
  DAMP_V_In/1 -> [DAMP_V]
  DAMP_T_In/1 -> [DAMP_T]
  DAMP_L_In/1 -> [DAMP_L]
  TEST_Y_In/1 -> [TEST_Y]
  TEST_P_In/1 -> [TEST_P]
  TEST_R_In/1 -> [TEST_R]
  TEST_V_In/1 -> [TEST_V]
  TEST_T_In/1 -> [TEST_T]
  TEST_L_In/1 -> [TEST_L]
  ISC_Y_In/1 -> [ISC_Y]
  ISC_P_In/1 -> [ISC_P]
  ISC_L_In/1 -> [ISC_L]
  OPTICALIGN_Y_In/1 -> [OPTICALIGN_Y]
  OPTICALIGN_P_In/1 -> [OPTICALIGN_P]
  Sum1/1 -> TRANS_MAIN_Out/1
  Sum2/1 -> VERT_MAIN_Out/1
  Sum5/1 -> ROLL_MAIN_Out/1
  [DAMP_L] -> Sum/3
  [TEST_L] -> Sum/2
  [ISC_L] -> Sum/1
  Sum/1 -> LONG_MAIN_Out/1
  Sum3/1 -> YAW_MAIN_Out/1
  Sum4/1 -> PITCH_MAIN_Out/1
  PSD_PIT/1 -> [PSD_PIT]
  PSD_YAW/1 -> [PSD_YAW]
  [PSD_PIT] -> Sum4/5
  [PSD_YAW] -> Sum3/5

== system PAYLOAD_MASTER/PAYLOADIM/ADDASC ==
  CAL_OSC_L_In : Inport
  CAL_EXC_L_In : Inport  Port=2
  ISC_L_In : Inport  Port=3
  ISC_P_In : Inport  Port=4
  ISC_Y_In : Inport  Port=5
  DITHER_P_In : Inport  Port=6
  DITHER_Y_In : Inport  Port=7
  OPLEV_L_In : Inport  Port=8
  OPLEV_P_In : Inport  Port=9
  OPLEV_Y_In : Inport  Port=10
  Sum1 : Sum  Inputs=++++
  Sum3 : Sum  Inputs=+++
  Sum4 : Sum  Inputs=+++
  LONG_Out : Outport
  PITCH_Out : Outport  Port=2
  YAW_Out : Outport  Port=3
  wires:
  OPLEV_Y_In/1 -> Sum3/3
  OPLEV_P_In/1 -> Sum4/3
  OPLEV_L_In/1 -> Sum1/4
  ISC_L_In/1 -> Sum1/3
  CAL_EXC_L_In/1 -> Sum1/2
  Sum1/1 -> LONG_Out/1
  CAL_OSC_L_In/1 -> Sum1/1
  DITHER_Y_In/1 -> Sum3/2
  DITHER_P_In/1 -> Sum4/2
  Sum4/1 -> PITCH_Out/1
  ISC_Y_In/1 -> Sum3/1
  ISC_P_In/1 -> Sum4/1
  Sum3/1 -> YAW_Out/1

== system PAYLOAD_MASTER/PAYLOADIM/ADD_LKIN ==
  LKN_V1_In : Inport
  LKN_V2_In : Inport  Port=2
  LKIN_V3_In : Inport  Port=3
  LKIN_H1_In : Inport  Port=4
  LKIN_H2_In : Inport  Port=5
  LKIN_H3_In : Inport  Port=6
  OSEM_V1_In : Inport  Port=7
  OSEM_V2_In : Inport  Port=8
  OSEM_V3_In : Inport  Port=9
  OSEM_H1_In : Inport  Port=10
  OSEM_H2_In : Inport  Port=11
  OSEM_H3_In : Inport  Port=12
  Sum{,1..5} (6 alike) : Sum
  V1_Out : Outport
  V2_Out : Outport  Port=2
  V3_Out : Outport  Port=3
  H1_Out : Outport  Port=4
  H2_Out : Outport  Port=5
  H3_Out : Outport  Port=6
  wires:
  LKIN_H3_In/1 -> Sum2/1
  LKIN_H2_In/1 -> Sum5/1
  Sum5/1 -> H2_Out/1
  OSEM_H2_In/1 -> Sum5/2
  Sum2/1 -> H3_Out/1
  OSEM_H3_In/1 -> Sum2/2
  LKIN_H1_In/1 -> Sum1/1
  LKIN_V3_In/1 -> Sum3/1
  LKN_V2_In/1 -> Sum4/1
  Sum/1 -> V1_Out/1
  LKN_V1_In/1 -> Sum/1
  OSEM_V1_In/1 -> Sum/2
  Sum3/1 -> V3_Out/1
  Sum4/1 -> V2_Out/1
  OSEM_V3_In/1 -> Sum3/2
  OSEM_V2_In/1 -> Sum4/2
  Sum1/1 -> H1_Out/1
  OSEM_H1_In/1 -> Sum1/2
